simulink model "operate-flexible-link"  (R2023a)
settings: Solver=ode4  StartTime=0.0  StopTime=15  FixedStep=1/30  RelTol=1e-3  EnableMultiTasking=on
undefined symbols (not defined in the file or in its folder): HIL
libraries: quarc_library x5, hostiolib x2, imaqlib x1
settings Model: SimulationMode=external  Creator=kentaroohki  LastModifiedBy=Flexible4
settings SolverCC: AlgebraicLoopSolver=TrustRegion  PositivePriorityOrder=on
settings DataIOCC: SaveOperatingPoint=on  SaveFormat=Structure  SaveOutput=off  SignalLogging=off  DSMLogging=off  InspectSignalLogs=on  SaveTime=off  ReturnWorkspaceOutputs=off
settings DebuggingCC: UnconnectedInputMsg=warning  UnconnectedOutputMsg=warning  UnconnectedLineMsg=warning  ArithmeticOperatorsInVariantConditions=warning
settings ModelReferenceCC: EnableRefExpFcnMdlSchedulingChecks=on
settings SFSimCC: SimUseLocalCustomCode=off  CustomCodeUndefinedFunction=UseInterfaceOnly
settings RTWCC: Description=QUARC Win64 Target Using Toolchain  SystemTargetFile=quarc_win64.tlc  TemplateMakefile=quarc_default_tmf  RTWUseLocalCustomCode=off  Toolchain=QUARC win64 | nmake (64-bit Windows)  BuildConfiguration=Faster Runs
settings STFCustomTargetCC: SystemTargetFile=quarc_win64.tlc
settings GRTTargetCC: ParMdlRefBuildCompliant=off  CompOptLevelCompliant=off  CombineOutputUpdateFcns=off  MatFileLogging=off  CPPClassGenCompliant=off  GRTInterface=on  ExtMode=on  ExtModeMexFile=quarc_comm

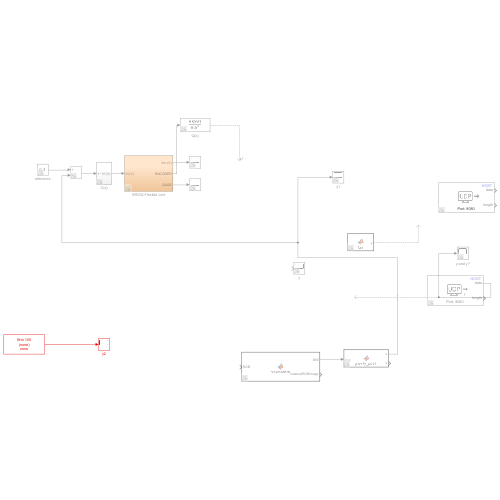
[thumbnail: Simulink's stored preview of the top-level diagram]
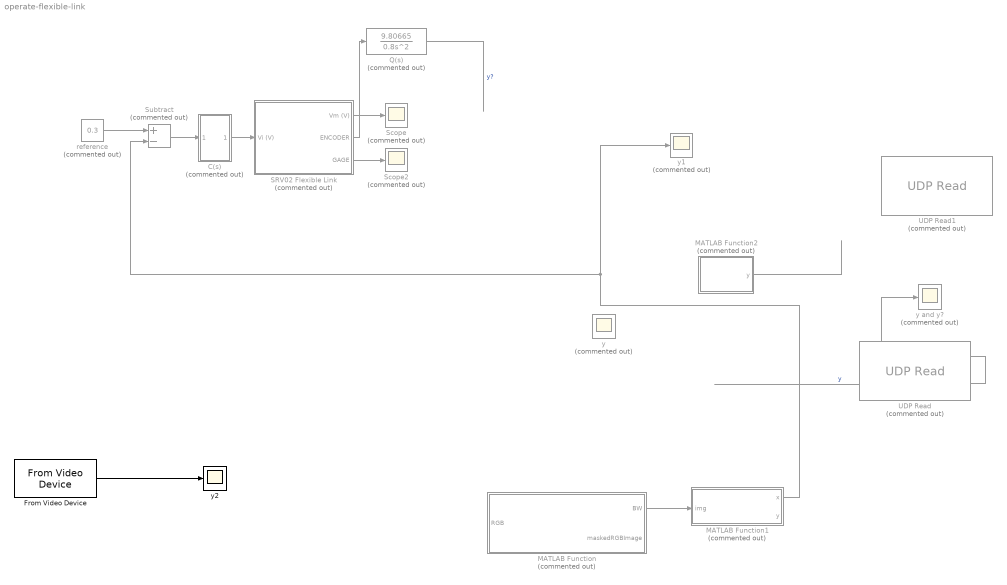
== system operate-flexible-link ==
  C(s) : Subsystem  Commented=on
  From Video Device : imaqlib/From Video Device  DeviceMenu=(none)  Device=winvideo 1 (Brio 100)  ObjConstructor=(none)  VideoFormatMenu=(none)  VideoFormat=(none)  VideoSource=none  ROIPosition=[0 0 576 1024]  EnableHWTrigger=off  SampleTime=1/30  OutputPortsMode=One multidimensional signal  DataType=double  CanDoHWTrigger=no  ReturnedColorSpace=rgb  BlockHandle=214.0002  ROIWidth=1024  ROIHeight=576  ROIColumn=0  ROIRow=0  EngXMLPath=C:\Program Files\MATLAB\R2023a\toolbox\imaq\imaq\private  DevXMLPath=C:\ProgramData\MATLAB\SupportPackages\R2023a\toolbox\imaq\supportpackages\genericvideo\adaptor\win64  EngLibPath=C:\Program Files\MATLAB\R2023a\toolbox\imaq\imaqblks\imaqmex\win64  ColorSpace=rgb  BayerSensorAlignment=grbg  ImaqMode=on
  MATLAB Function : MATLAB Function  Commented=on  TreatAsAtomicUnit=on
  MATLAB Function1 : MATLAB Function  Commented=on  TreatAsAtomicUnit=on
  MATLAB Function2 : MATLAB Function  Commented=on  TreatAsAtomicUnit=on
  Q(s) : TransferFcn  Commented=on  Numerator=[9.80665]  Denominator=[0.8 0 0]
  SRV02 Flexible Link : Subsystem  Commented=on
  Scope : Scope  Commented=on
  Scope2 : Scope  Commented=on
  Subtract : Sum  Commented=on  Inputs=+-
  UDP Read : hostiolib/UDP Read  Commented=on  localURL='0.0.0.0'  localPort=8080  remoteURL='0.0.0.0'  remotePort=-1  recvBufferSize=8192  dims=1  signalDatatype=double  isVarSize=off  showBlockingTime=on  blockingTime=1/30  sampletime=1/30  blockPlatform=HOST  hoistedMaskSrc=UDP Read/UDP Read Sim/UDP Read
  UDP Read1 : hostiolib/UDP Read  Commented=on  localURL='0.0.0.0'  localPort=8080  remoteURL='0.0.0.0'  remotePort=-1  recvBufferSize=8192  dims=1  signalDatatype=double  isVarSize=off  showBlockingTime=on  blockingTime=1/30  sampletime=1/30  blockPlatform=HOST  hoistedMaskSrc=UDP Read/UDP Read Sim/UDP Read
  reference : Constant  Commented=on  Value=0.3
  y : Scope  Commented=on
  y and y? : Scope  Commented=on
  y1 : Scope  Commented=on
  y2 : Scope
  wires:
  C(s)/1(Vi (V)) -> SRV02 Flexible Link/1(Vi (V))
  SRV02 Flexible Link/2(ENCODER) -> Q(s)/1
  SRV02 Flexible Link/3(GAGE) -> Scope2/1
  SRV02 Flexible Link/1(Vm (V)) -> Scope/1
  UDP Read/1 -> y and y?/1  "y"
  Q(s)/1 -> ?  "y?"
  reference/1 -> Subtract/1
  Subtract/1 -> C(s)/1(In1)
  MATLAB Function1/1(x) -> y1/1, Subtract/2
  From Video Device/1 -> y2/1
  MATLAB Function/1(BW) -> MATLAB Function1/1(img)
  MATLAB Function2/1(y) -> ?

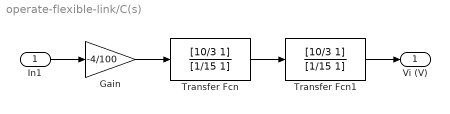
== system operate-flexible-link/C(s) ==
  In1 : Inport
  Gain : Gain  Gain=-4/100
  Transfer Fcn : TransferFcn  Numerator=[10/3 1]  Denominator=[1/15 1]
  Transfer Fcn1 : TransferFcn  Numerator=[10/3 1]  Denominator=[1/15 1]
  Vi (V) : Outport
  wires:
  Transfer Fcn/1 -> Transfer Fcn1/1
  Transfer Fcn1/1 -> Vi (V)/1
  Gain/1 -> Transfer Fcn/1
  In1/1 -> Gain/1

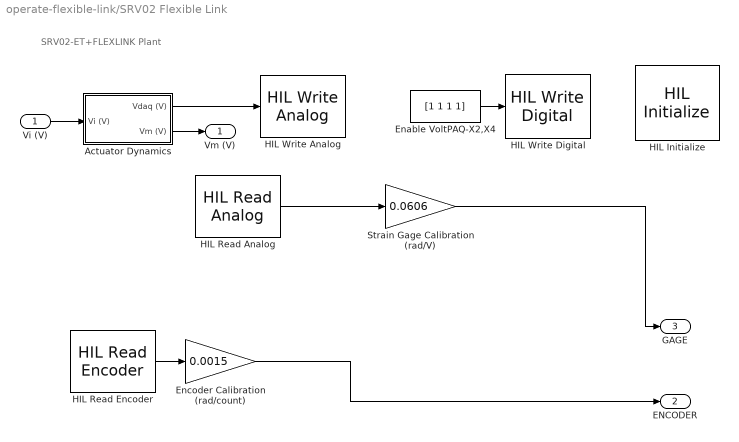
== system operate-flexible-link/SRV02 Flexible Link ==
  note: SRV02-ET+FLEXLINK Plant
  Vi (V) : Inport
  Actuator Dynamics : Subsystem
  Enable VoltPAQ-X2,X4 : Constant  Value=[1 1 1 1]
  Encoder Calibration (rad/count) : Gain  Gain=0.0015  SaturateOnIntegerOverflow=on  OutDataTypeStr=Inherit: Same as input  ParamDataTypeStr=Inherit: Same as input
  HIL Initialize : quarc_library/Data Acquisition/Generic/Configuration/HIL Initialize  object_name=HIL-1  board_type=q2_usb  board_number=0  board_options=d0=digital;d1=digital;led=auto;update_rate=normal  exclusive=off  active=off  hardware_clocks=[0:2]  clock_modes=[]  initial_clock_frequencies=[]  set_clock_params_at_start=off  set_clock_params_at_switch_in=off  set_clock_frequencies_at_start=off  set_clock_frequencies_at_switch_in=off  analog_input_channels=[0:1]  analog_input_configurations=[]  analog_input_maximums=10  analog_input_minimums=-10  set_analog_input_params_at_start=on  set_analog_input_params_at_switch_in=off  analog_output_channels=[0:1]  analog_output_maximums=10  analog_output_minimums=-10  initial_analog_outputs=[0]  final_analog_outputs=[0]  watchdog_analog_outputs=0  set_analog_output_params_at_start=on  set_analog_output_params_at_switch_in=off  set_analog_outputs_at_start=on  set_analog_outputs_at_switch_in=off  set_analog_outputs_at_terminate=on  set_analog_outputs_at_switch_out=off  set_analog_outputs_on_watchdog=off  digital_input_channels=[]  digital_output_channels=[0:7]  digital_output_configuration=[]  initial_digital_outputs=[0]  final_digital_outputs=[0]  watchdog_digital_outputs=[0]  set_digital_output_params_at_start=off  set_digital_output_params_at_switch_in=off  set_digital_outputs_at_start=on  set_digital_outputs_at_switch_in=off  set_digital_outputs_at_terminate=on  set_digital_outputs_at_switch_out=off  set_digital_outputs_on_watchdog=off  encoder_channels=[0:1]  quadrature=[4]  encoder_filter_frequency=[]  initial_encoder_counts=[0]  set_encoder_params_at_start=on  set_encoder_params_at_switch_in=off  set_encoder_counts_at_start=on  set_encoder_counts_at_switch_in=off  pwm_channels=[]  pwm_modes=[0]  pwm_frequency=1/0.020  pwm_configuration=[]  pwm_alignment=[]  pwm_polarity=[]  pwm_leading_deadband=[]  pwm_trailing_deadband=[]  initial_pwm_outputs=[0]  final_pwm_outputs=[0]  watchdog_pwm_outputs=[0]  set_pwm_params_at_start=on  set_pwm_params_at_switch_in=off  set_pwm_outputs_at_start=on  set_pwm_outputs_at_switch_in=off  set_pwm_outputs_at_terminate=on  set_pwm_outputs_at_switch_out=off  set_pwm_outputs_on_watchdog=off  other_output_channels=[]  initial_other_outputs=[]  final_other_outputs=[]  watchdog_other_outputs=[]  set_other_outputs_at_start=off  set_other_outputs_at_switch_in=off  set_other_outputs_at_terminate=off  set_other_outputs_at_switch_out=off  set_other_outputs_on_watchdog=off
  HIL Read Analog : quarc_library/Data Acquisition/Generic/Immediate I//O/HIL Read Analog  object_name=HIL-1  channels=0  sample_time=qc_get_step_size  active=on  vector_output=off
  HIL Read Encoder : quarc_library/Data Acquisition/Generic/Immediate I//O/HIL Read Encoder  object_name=HIL-1  channels=0  sample_time=qc_get_step_size  active=on  vector_output=off  data_type_mode=Inherit via back propagation  data_type=double
  HIL Write Analog : quarc_library/Data Acquisition/Generic/Immediate I//O/HIL Write Analog  object_name=HIL-1  channels=0  sample_time=-1  active=off  vector_input=off
  HIL Write Digital : quarc_library/Data Acquisition/Generic/Immediate I//O/HIL Write Digital  object_name=HIL-1  channels=[0:3]  sample_time=-1  active=off  vector_input=on
      settings: SourceProductName=QUARC Targets
  Strain Gage Calibration (rad/V) : Gain  Gain=0.0606  SaturateOnIntegerOverflow=on  OutDataTypeStr=Inherit: Same as input  ParamDataTypeStr=Inherit: Same as input
  Vm (V) : Outport  InitialOutput=0  VectorParamsAs1DForOutWhenUnconnected=off
  ENCODER : Outport  Port=2  InitialOutput=0  VectorParamsAs1DForOutWhenUnconnected=off
  GAGE : Outport  Port=3  InitialOutput=0  VectorParamsAs1DForOutWhenUnconnected=off
  wires:
  Encoder Calibration (rad/count)/1 -> ENCODER/1
  Actuator Dynamics/2(Vm (V)) -> Vm (V)/1
  Actuator Dynamics/1(Vdaq (V)) -> HIL Write Analog/1
  Vi (V)/1 -> Actuator Dynamics/1(Vi (V))
  Enable VoltPAQ-X2,X4/1 -> HIL Write Digital/1
  HIL Read Analog/1 -> Strain Gage Calibration (rad/V)/1
  Strain Gage Calibration (rad/V)/1 -> GAGE/1
  HIL Read Encoder/1 -> Encoder Calibration (rad/count)/1

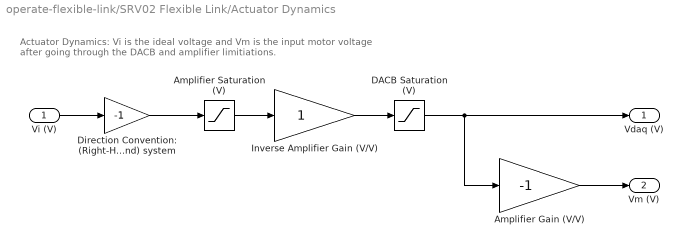
== system operate-flexible-link/SRV02 Flexible Link/Actuator Dynamics ==
  note: Actuator Dynamics: Vi is the ideal voltage and Vm is the
      | input motor voltage after going through the DACB and amplifier limitiations.
  Vi (V) : Inport
  Amplifier Saturation (V) : Saturate  UpperLimit=24  LowerLimit=-24
  Amplifier Gain (V/V) : Gain  Gain=-1
  DACB Saturation (V) : Saturate  UpperLimit=10  LowerLimit=-10
  Direction Convention: (Right-Hand) system : Gain  Gain=-1  SaturateOnIntegerOverflow=on  OutDataTypeStr=Inherit: Same as input  ParamDataTypeStr=Inherit: Same as input
  Inverse Amplifier Gain (V/V) : Gain
  Vdaq (V) : Outport  VectorParamsAs1DForOutWhenUnconnected=off
  Vm (V) : Outport  Port=2  VectorParamsAs1DForOutWhenUnconnected=off
  wires:
  Direction Convention: (Right-Hand) system/1 -> Amplifier Saturation (V)/1
  Amplifier Gain (V/V)/1 -> Vm (V)/1
  DACB Saturation (V)/1 -> Vdaq (V)/1, Amplifier Gain (V/V)/1
  Inverse Amplifier Gain (V/V)/1 -> DACB Saturation (V)/1
  Amplifier Saturation (V)/1 -> Inverse Amplifier Gain (V/V)/1
  Vi (V)/1 -> Direction Convention: (Right-Hand) system/1

== matlab function operate-flexible-link/MATLAB Function ==
  data: RGB input; BW output; maskedRGBImage output
function [BW, maskedRGBImage] = createMask(RGB)
%createMask  Threshold RGB image using auto-generated code from colorThresholder app.
%  [BW,MASKEDRGBIMAGE] = createMask(RGB) thresholds image RGB using
%  auto-generated code from the colorThresholder app. The colorspace and
%  range for each channel of the colorspace were set within the app. The
%  segmentation mask is returned in BW, and a composite of the mask and
%  original RGB images is returned in maskedRGBImage.

% Auto-generated by colorThresholder app on 07-May-2026
%------------------------------------------------------


% Convert RGB image to chosen color space
I = rgb2hsv(RGB);

% Define thresholds for channel 1 based on histogram settings
channel1Min = 0;
channel1Max = 80/255;

% Define thresholds for channel 2 based on histogram settings
channel2Min = 90/255;
channel2Max = 1;

% Define thresholds for channel 3 based on histogram settings
channel3Min = 100/255;
channel3Max = 1;

% Create mask based on chosen histogram thresholds
sliderBW = (I(:,:,1) >= channel1Min ) & (I(:,:,1) <= channel1Max) & ...
    (I(:,:,2) >= channel2Min ) & (I(:,:,2) <= channel2Max) & ...
    (I(:,:,3) >= channel3Min ) & (I(:,:,3) <= channel3Max);
BW = sliderBW;

% Initialize output masked image based on input image.
maskedRGBImage = RGB;

% Set background pixels where BW is false to zero.
maskedRGBImage(repmat(~BW,[1 1 3])) = 0;

end

== matlab function operate-flexible-link/MATLAB Function2 ==
  data: y output
function y = fcn()

y = pyrunfile("ref_once.py","x");

== matlab function operate-flexible-link/MATLAB Function1 ==
  data: x output; img input; y output
function [x,y] = gravity_point(img)
[x_size, y_size] = size(img);
x_pos = 1:x_size;
y_pos = 1:y_size;

x_all = 0;
y_all = 0;

for i = y_pos
    x_all = x_all + sum((img(:,i) .* (x_pos)'))/sum(img(:,i));
end
x = mean(x_all)/x_size;

for i = x_pos
    y_all = y_all + sum((img(i,:) .* (y_pos)'))/sum(img(i,:));
end
y = mean(y_all)/y_size;

end
